simulink model "dcmotor_controller"  (Simulink 7.8)
settings: Solver=FixedStepDiscrete  StartTime=0.0  StopTime=10.0  RelTol=1e-3
undefined symbols (not defined in the file): Down, Up
libraries: tiiqmathlib x4, c28xdmclib x4, c280xlib x3, idelinklib_ticcs x1, idelinklib_tgtpref x1
settings Model: Creator=hardware  LastModifiedBy=kuba
settings DataIOCC: SaveOutput=off  SaveTime=off
settings OptimizationCC: OptimizeModelRefInitCode=on  LifeSpan=1
settings HardwareCC: ProdBitPerChar=16  ProdBitPerInt=16  ProdBitPerPointer=16  ProdLargestAtomicInteger=Integer  ProdIntDivRoundTo=Zero  ProdEndianess=LittleEndian  ProdWordSize=16  ProdHWDeviceType=Texas Instruments->C2000
settings RTWCC: SystemTargetFile=idelink_ert.tlc  GenerateMakefile=off  TemplateMakefile=idelink_ert.tmf  Description=IDE Link ERT  ProcessScript=idelink_ert_make_rtw_hook
settings CodeAppCC: IgnoreCustomStorageClasses=off
settings ERTFactory: TargetFcnLib=ansi_tfl_table_tmw.mat  TargetFunctionLibrary=ANSI_C  UtilityFuncGeneration=Auto  ERTMultiwordTypeDef=System defined  CodeExecutionProfiling=off  ERTMultiwordLength=256  MultiwordLength=2048  GenerateFullHeader=on  GenerateSampleERTMain=off  GenerateTestInterfaces=off  IsPILTarget=off  ModelReferenceCompliant=on  ParMdlRefBuildCompliant=off  CompOptLevelCompliant=off  ConcurrentExecutionCompliant=on  IncludeMdlTerminateFcn=on  GeneratePreprocessorConditionals=Disable all  CombineOutputUpdateFcns=on  CombineSignalStateStructs=off  SuppressErrorStatus=off  ERTFirstTimeCompliant=on  IncludeFileDelimiter=Auto  ERTCustomFileBanners=on  SupportAbsoluteTime=on  LogVarNameModifier=rt_  MatFileLogging=off  MultiInstanceERTCode=off  SupportNonFinite=on  SupportComplex=on  PurelyIntegerCode=off  SupportContinuousTime=off  SupportNonInlinedSFcns=off  SupportVariableSizeSignals=off  EnableShiftOperators=on  ParenthesesLevel=Nominal  PortableWordSizes=off  ModelStepFunctionPrototypeControlCompliant=on  CPPClassGenCompliant=off  AutosarCompliant=off  GenerateErtSFunction=off  CreateSILPILBlock=None  CodeExecutionProfileVariable=executionProfile  CodeProfilingSaveOptions=SummaryOnly  GenerateASAP2=off  ExtMode=off  ExtModeTransport=0  ExtModeStaticAlloc=off  ExtModeStaticAllocSize=1000000  ExtModeTesting=off  ExtModeMexFile=TIC2000ExternalModeOpen  ExtModeIntrfLevel=Level2 - Open  InlinedParameterPlacement=Hierarchical  TargetOS=BareBoardExample  MultiInstanceErrorCode=Error  RateGroupingCode=on  RootIOFormat=Individual arguments  RTWCAPISignals=off  RTWCAPIParams=off  RTWCAPIStates=off  RTWCAPIRootIO=off  ERTSrcFileBannerTemplate=ert_code_template.cgt  ERTHdrFileBannerTemplate=ert_code_template.cgt  ERTDataSrcFileTemplate=ert_code_template.cgt  ERTDataHdrFileTemplate=ert_code_template.cgt  ERTCustomFileTemplate=example_file_process.tlc  CoverageDialogOpen=off  EnableDataOwnership=off  SignalDisplayLevel=10  ParamTuneLevel=10  GlobalDataDefinition=Auto  DataDefinitionFile=global.c  GlobalDataReference=Auto  ERTFilePackagingFormat=Modular  DataReferenceFile=global.h  GRTInterface=off  PreserveExpressionOrder=off  PreserveIfCondition=off  ConvertIfToSwitch=off  PreserveExternInFcnDecls=on  SuppressUnreachableDefaultCases=off  EnableUserReplacementTypes=off  MemSecPackage=--- None ---  MemSecDataConstants=Default  MemSecDataIO=Default  MemSecDataInternal=Default  MemSecDataParameters=Default  MemSecFuncInitTerm=Default  MemSecFuncExecute=Default  MemSecFuncSharedUtil=Default  CodeProfilingInstrumentation=off  AdaptorName=Texas Instruments Code Composer Studio  exportIDEObj=on  ideObjName=IDE_Obj  oldideObjName=IDE_Obj  ideObjTimeout=10  oldideObjTimeout=10  ideObjBuildTimeout=1000  oldideObjBuildTimeout=1000  ProfileGenCode=off  profileBy=Tasks  ProfileNumSamples=100  InlineDSPBlks=off  projectOptions=Custom  debugCompilerOptions="-g -D\"_DEBUG\""  releaseCompilerOptions=-o2  getCompilerOptions=off  resetCompilerOptions=off  getLinkerOptions=off  resetLinkerOptions=off  systemStackSize=512  systemHeapSize=512  buildFormat=Project  buildAction=Build_and_execute  overrunNotificationMethod=None  overrunNotificationFcn=myfunction  oldoverrunNotificationFcn=myfunction  configurePIL=off  configPILBlockAction=Create_PIL_block_build_and_download  DiagnosticActions=warning

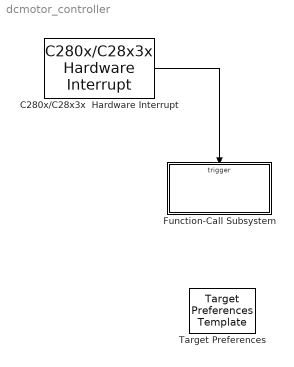
== system dcmotor_controller ==
  C280x/C28x3x  Hardware Interrupt : idelinklib_ticcs/C280x//C28x3x Hardware Interrupt  irqnumbers=[3]  pienumbers=[1]  irqpriorities=[30]  irqpreempts=[0]  showinput=off  dspchiptype=C280X
  Function-Call Subsystem : Subsystem  TreatAsAtomicUnit=on
  Target Preferences : idelinklib_tgtpref/Target Preferences Template  Tag=ccslinktgtpref  library=off
  wires:
  C280x/C28x3x  Hardware Interrupt/1 -> Function-Call Subsystem/Trigger

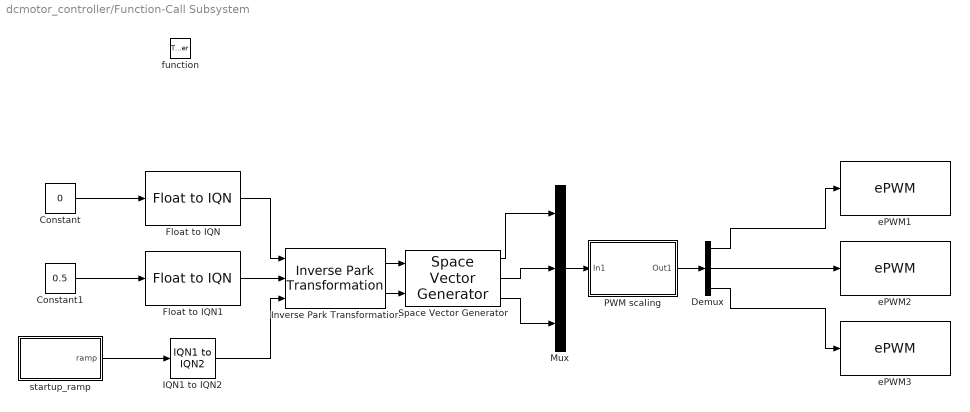
== system dcmotor_controller/Function-Call Subsystem ==
  function : TriggerPort  TriggerType=function-call
  Constant : Constant  Value=0  OutDataTypeStr=single
  Constant1 : Constant  Value=0.5  OutDataTypeStr=single
  Demux : Demux  Outputs=3
  Float to IQN : tiiqmathlib/Float to IQN  Q_value=24
  Float to IQN1 : tiiqmathlib/Float to IQN  Q_value=24
  IQN1 to IQN2 : tiiqmathlib/IQN1 to IQN2  New_Q=24
  Inverse Park Transformation : c28xdmclib/Inverse Park Transformation
  Mux : Mux  Inputs=3
  PWM scaling : Subsystem
  Space Vector Generator : c28xdmclib/Space Vector Generator
  ePWM1 : c280xlib/ePWM  checkMode=off  useModule=ePWM1  periodUnits=Clock cycles  timerSource=Specify via dialog  timerPeriod_clk=(2^12)+1  timerPeriod_sec=0.0001  countingMode=Up-Down  synchronizationOption=Disable  synchronizationEnable=off  phaseActiveEnable=Disable  phaseDirection=Count down after sync  phaseActive=0  clockPrescale=1  HSclockPrescale=1  ePWMxAStatus=on  CMPAUnits=Clock cycles  CMPASource=Input port  CMPAValue_per=50  CMPAValue_clk=5000  ePWMxAactionLogic1=Do nothing  ePWMxAactionLogic2=Do nothing  ePWMxAactionLogic3=Set  ePWMxAactionLogic4=Clear  ePWMxAactionLogic5=Do nothing  ePWMxAactionLogic6=Do nothing  ePWMxALoadMode=Load on CTR=Zero  ePWMxACSFenable=off  ePWMxACSFvalue=Forcing Disable  ePWMxASFreload=Zero  enHRPWM=off  HRPWM_LoadMode=CTR=ZERO  HRPWM_CTLMode=Phase control mode  HRPWM_EDGMode=Both edge  enSFO=on  ePWMxBStatus=off  CMPBUnits=Clock cycles  CMPBSource=Specify via dialog  CMPBValue_per=0  CMPBValue_clk=0  ePWMxBactionLogic1=Do nothing  ePWMxBactionLogic2=Do nothing  ePWMxBactionLogic3=Do nothing  ePWMxBactionLogic4=Do nothing  ePWMxBactionLogic5=Do nothing  ePWMxBactionLogic6=Do nothing  ePWMxBLoadMode=Load on CTR=Zero  ePWMxBCSFenable=off  ePWMxBCSFvalue=Forcing Disable  ePWMxBSFreload=Zero  enableDBePWMxA=on  enableDBePWMxB=on  DBpolarity=AHC  DBedgeDelay=Positive  DBSource_ePWMxA=ePWMxA  DBSource_ePWMxB=ePWMxA  DBperiodSource=Specify via dialog  REDperiod=15  FEDperiod=15  adcstartModuleA=on  adcrequestEventA=First event  adcstartEventA=CTR=Zero  adcstartModuleB=off  adcrequestEventB=First event  adcstartEventB=CTR=Zero  intEn=on  intPrd=First event  intSel=CTR=Zero  chopperEnable=off  chopperFrequency=1  chopperFirstwidth=1  chopperDuty=12.5%  tripZonesource=Specify via dialog  tzselOSHT1=off  tzselOSHT2=off  tzselOSHT3=off  tzselOSHT4=off  tzselOSHT5=off  tzselOSHT6=off  tzselCBC1=off  tzselCBC2=off  tzselCBC3=off  tzselCBC4=off  tzselCBC5=off  tzselCBC6=off  enTzOstIntr=off  enTzCbcIntr=off  ePWMxAforced=No action  ePWMxBforced=No action  timerPeriod=-1  ePWMxAValue=1  ePWMxBValue=0  tripZoneoption=OSHT
  ePWM2 : c280xlib/ePWM  checkMode=off  useModule=ePWM2  periodUnits=Clock cycles  timerSource=Specify via dialog  timerPeriod_clk=(2^12)+1  timerPeriod_sec=0.0001  countingMode=Up-Down  synchronizationOption=Disable  synchronizationEnable=off  phaseActiveEnable=Disable  phaseDirection=Count down after sync  phaseActive=0  clockPrescale=1  HSclockPrescale=1  ePWMxAStatus=on  CMPAUnits=Clock cycles  CMPASource=Input port  CMPAValue_per=50  CMPAValue_clk=5000  ePWMxAactionLogic1=Do nothing  ePWMxAactionLogic2=Do nothing  ePWMxAactionLogic3=Set  ePWMxAactionLogic4=Clear  ePWMxAactionLogic5=Do nothing  ePWMxAactionLogic6=Do nothing  ePWMxALoadMode=Load on CTR=Zero  ePWMxACSFenable=off  ePWMxACSFvalue=Forcing Disable  ePWMxASFreload=Zero  enHRPWM=off  HRPWM_LoadMode=CTR=ZERO  HRPWM_CTLMode=Phase control mode  HRPWM_EDGMode=Both edge  enSFO=on  ePWMxBStatus=off  CMPBUnits=Clock cycles  CMPBSource=Specify via dialog  CMPBValue_per=0  CMPBValue_clk=0  ePWMxBactionLogic1=Do nothing  ePWMxBactionLogic2=Do nothing  ePWMxBactionLogic3=Do nothing  ePWMxBactionLogic4=Do nothing  ePWMxBactionLogic5=Do nothing  ePWMxBactionLogic6=Do nothing  ePWMxBLoadMode=Load on CTR=Zero  ePWMxBCSFenable=off  ePWMxBCSFvalue=Forcing Disable  ePWMxBSFreload=Zero  enableDBePWMxA=on  enableDBePWMxB=on  DBpolarity=AHC  DBedgeDelay=Positive  DBSource_ePWMxA=ePWMxA  DBSource_ePWMxB=ePWMxA  DBperiodSource=Specify via dialog  REDperiod=15  FEDperiod=15  adcstartModuleA=off  adcrequestEventA=First event  adcstartEventA=CTR=Zero  adcstartModuleB=off  adcrequestEventB=First event  adcstartEventB=CTR=Zero  intEn=off  intPrd=First event  intSel=CTR=Zero  chopperEnable=off  chopperFrequency=1  chopperFirstwidth=1  chopperDuty=12.5%  tripZonesource=Specify via dialog  tzselOSHT1=off  tzselOSHT2=off  tzselOSHT3=off  tzselOSHT4=off  tzselOSHT5=off  tzselOSHT6=off  tzselCBC1=off  tzselCBC2=off  tzselCBC3=off  tzselCBC4=off  tzselCBC5=off  tzselCBC6=off  enTzOstIntr=off  enTzCbcIntr=off  ePWMxAforced=No action  ePWMxBforced=No action  timerPeriod=-1  ePWMxAValue=1  ePWMxBValue=0  tripZoneoption=OSHT
  ePWM3 : c280xlib/ePWM  checkMode=off  useModule=ePWM3  periodUnits=Clock cycles  timerSource=Specify via dialog  timerPeriod_clk=(2^12)+1  timerPeriod_sec=0.0001  countingMode=Up-Down  synchronizationOption=Disable  synchronizationEnable=off  phaseActiveEnable=Disable  phaseDirection=Count down after sync  phaseActive=0  clockPrescale=1  HSclockPrescale=1  ePWMxAStatus=on  CMPAUnits=Clock cycles  CMPASource=Input port  CMPAValue_per=50  CMPAValue_clk=5000  ePWMxAactionLogic1=Do nothing  ePWMxAactionLogic2=Do nothing  ePWMxAactionLogic3=Set  ePWMxAactionLogic4=Clear  ePWMxAactionLogic5=Do nothing  ePWMxAactionLogic6=Do nothing  ePWMxALoadMode=Load on CTR=Zero  ePWMxACSFenable=off  ePWMxACSFvalue=Forcing Disable  ePWMxASFreload=Zero  enHRPWM=off  HRPWM_LoadMode=CTR=ZERO  HRPWM_CTLMode=Phase control mode  HRPWM_EDGMode=Both edge  enSFO=on  ePWMxBStatus=off  CMPBUnits=Clock cycles  CMPBSource=Specify via dialog  CMPBValue_per=0  CMPBValue_clk=0  ePWMxBactionLogic1=Do nothing  ePWMxBactionLogic2=Do nothing  ePWMxBactionLogic3=Do nothing  ePWMxBactionLogic4=Do nothing  ePWMxBactionLogic5=Do nothing  ePWMxBactionLogic6=Do nothing  ePWMxBLoadMode=Load on CTR=Zero  ePWMxBCSFenable=off  ePWMxBCSFvalue=Forcing Disable  ePWMxBSFreload=Zero  enableDBePWMxA=on  enableDBePWMxB=on  DBpolarity=AHC  DBedgeDelay=Positive  DBSource_ePWMxA=ePWMxA  DBSource_ePWMxB=ePWMxA  DBperiodSource=Specify via dialog  REDperiod=15  FEDperiod=15  adcstartModuleA=off  adcrequestEventA=First event  adcstartEventA=CTR=Zero  adcstartModuleB=off  adcrequestEventB=First event  adcstartEventB=CTR=Zero  intEn=off  intPrd=First event  intSel=CTR=Zero  chopperEnable=off  chopperFrequency=1  chopperFirstwidth=1  chopperDuty=12.5%  tripZonesource=Specify via dialog  tzselOSHT1=off  tzselOSHT2=off  tzselOSHT3=off  tzselOSHT4=off  tzselOSHT5=off  tzselOSHT6=off  tzselCBC1=off  tzselCBC2=off  tzselCBC3=off  tzselCBC4=off  tzselCBC5=off  tzselCBC6=off  enTzOstIntr=off  enTzCbcIntr=off  ePWMxAforced=No action  ePWMxBforced=No action  timerPeriod=-1  ePWMxAValue=1  ePWMxBValue=0  tripZoneoption=OSHT
  startup_ramp : Subsystem
  wires:
  Inverse Park Transformation/1 -> Space Vector Generator/1
  Inverse Park Transformation/2 -> Space Vector Generator/2
  Space Vector Generator/1 -> Mux/1
  Space Vector Generator/2 -> Mux/2
  Space Vector Generator/3 -> Mux/3
  PWM scaling/1(Out1) -> Demux/1
  Mux/1 -> PWM scaling/1(In1)
  Demux/1 -> ePWM1/1
  Demux/2 -> ePWM2/1
  Demux/3 -> ePWM3/1
  Float to IQN/1 -> Inverse Park Transformation/1
  Float to IQN1/1 -> Inverse Park Transformation/2
  Constant/1 -> Float to IQN/1
  Constant1/1 -> Float to IQN1/1
  startup_ramp/1(ramp) -> IQN1 to IQN2/1
  IQN1 to IQN2/1 -> Inverse Park Transformation/3

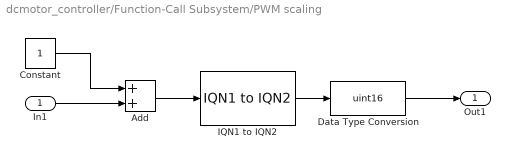
== system dcmotor_controller/Function-Call Subsystem/PWM scaling ==
  In1 : Inport
  Add : Sum
  Constant : Constant  OutDataTypeStr=fixdt(1,32,17)
  Data Type Conversion : DataTypeConversion  OutDataTypeStr=uint16  ConvertRealWorld=Stored Integer (SI)
  IQN1 to IQN2 : tiiqmathlib/IQN1 to IQN2  New_Q=11
  Out1 : Outport
  wires:
  IQN1 to IQN2/1 -> Data Type Conversion/1
  Constant/1 -> Add/1
  Add/1 -> IQN1 to IQN2/1
  Data Type Conversion/1 -> Out1/1
  In1/1 -> Add/2

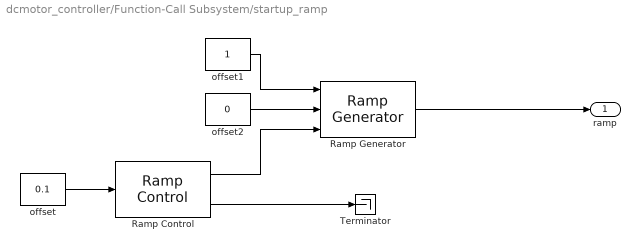
== system dcmotor_controller/Function-Call Subsystem/startup_ramp ==
  Ramp Control : c28xdmclib/Ramp Control  rmp_dly_max=1  rmp_lo_limit=0  rmp_hi_limit=1
  Ramp Generator : c28xdmclib/Ramp Generator  step_angle_max=0.005
  Terminator : Terminator
  offset : Constant  Value=0.1  OutDataTypeStr=fixdt(1,32,17)  SampleTime=-1
  offset1 : Constant  OutDataTypeStr=fixdt(1,32,17)  SampleTime=-1
  offset2 : Constant  Value=0  OutDataTypeStr=fixdt(1,32,17)  SampleTime=-1
  ramp : Outport
  wires:
  Ramp Control/1 -> Ramp Generator/3
  offset/1 -> Ramp Control/1
  Ramp Control/2 -> Terminator/1
  offset2/1 -> Ramp Generator/2
  offset1/1 -> Ramp Generator/1
  Ramp Generator/1 -> ramp/1
